simulink model "saturated_control_control101"  (R2024a)
settings: Solver=VariableStepAuto  StartTime=0.0  StopTime=20  RelTol=1e-3
undefined symbols (not defined in the file or in its folder): umax, umin
libraries: cstblocks x1
settings Model: Creator=barsr  LastModifiedBy=Anthony Rossiter
settings RTWCC: GPUComputeCapability=3.5

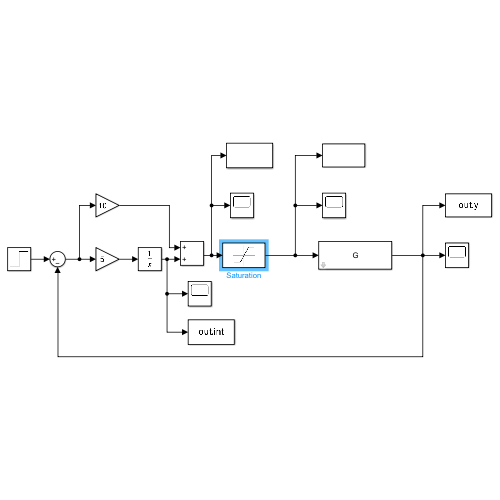
[thumbnail: Simulink's stored preview of the top-level diagram]
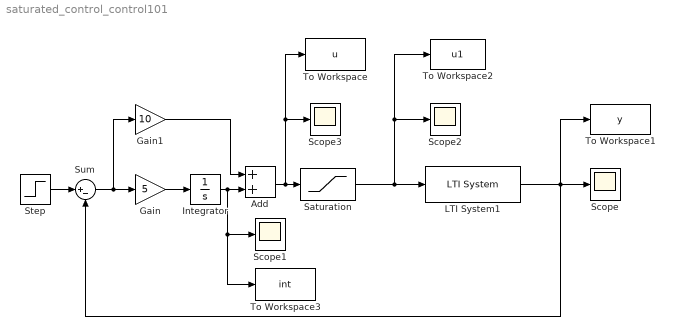
== system saturated_control_control101 ==
  Add : Sum
  Gain : Gain  Gain=5
  Gain1 : Gain  Gain=10
  Integrator : Integrator
  LTI System1 : cstblocks/LTI System  sys=G  IC=[]  PadeOrder=0
  Saturation : Saturate  UpperLimit=umax  LowerLimit=umin
  Scope{,1..3} (4 alike) : Scope
  Step : Step  Time=0  SampleTime=0
  Sum : Sum  Inputs=|+-
  To Workspace : ToWorkspace  VariableName=u  SaveFormat=Structure With Time  SampleTime=-1
  To Workspace1 : ToWorkspace  VariableName=y  SaveFormat=Structure With Time  SampleTime=-1
  To Workspace2 : ToWorkspace  VariableName=u1  SaveFormat=Structure With Time  SampleTime=-1
  To Workspace3 : ToWorkspace  VariableName=int  SaveFormat=Structure With Time  SampleTime=-1
  wires:
  Step/1 -> Sum/1
  Saturation/1 -> LTI System1/1, To Workspace2/1, Scope2/1
  LTI System1/1 -> Sum/2, Scope/1, To Workspace1/1
  Gain/1 -> Integrator/1
  Sum/1 -> Gain/1, Gain1/1
  Integrator/1 -> To Workspace3/1, Scope1/1, Add/2
  Add/1 -> To Workspace/1, Scope3/1, Saturation/1
  Gain1/1 -> Add/1
